simulink model "test_mashinka_mapp_4"  (R2020b)
settings: Solver=ode45  StartTime=0.0  StopTime=20000  RelTol=1e-3  EnableMultiTasking=on
undefined symbols (not defined in the file): CMD_ci_Re_9, CMD_fb, CMD_Firprg_0, CMD_Firprg_1, CMD_gain, CMD_ind_mult, CMD_ind_mult_1, CMD_ind_mult_2, CMD_ind_mult_3, CMD_ind_mult_4, CMD_ind_vol, CMD_ind_vol_1, CMD_ind_vol_2, CMD_ind_vol_3, CMD_ind_vol_4, CMD_nl, CMD_param_0, CMD_pedal, CMD_reset, CMD_shape_0, CMD_step_down, CMD_step_up, ind_mult_0, ind_mult_1, ind_mult_2, ind_mult_3, ind_mult_4, ind_mult_multiplier, num_harm_0, num_pts0, num_str0, num_str1, Res, rom_length
libraries: xbsIndex_r4 x2299
(part 6 of 11)

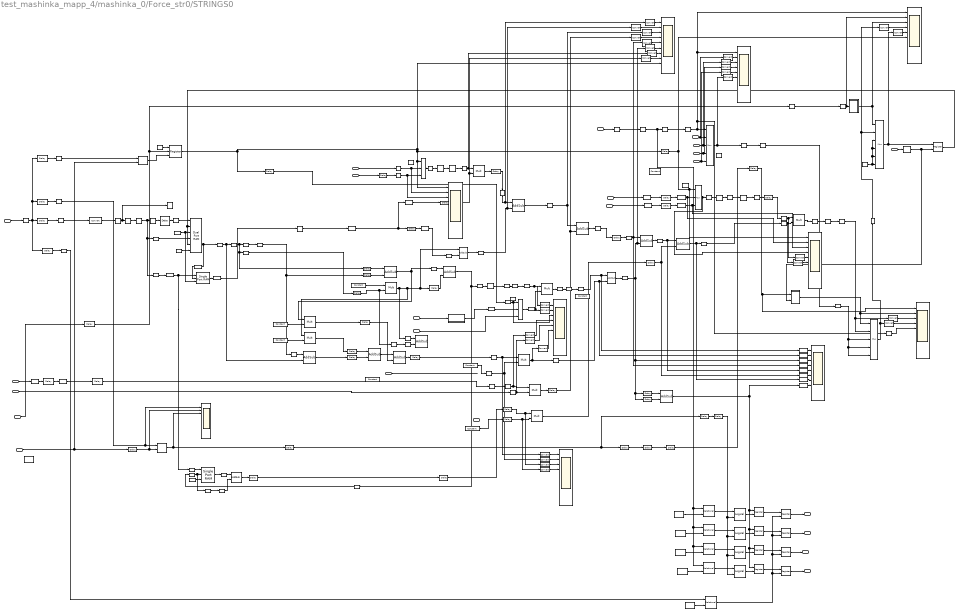
== system test_mashinka_mapp_4/mashinka_0/Force_str0/STRINGS0 ==
  note: Str1[i-2] + Str1[i+2]
  note: 6*Str1[i]
  note: next_plus_last
  note: ff
  note: w20
  note: w41
  note: curr
  note: next
  note: last
  note: prev
  note: decr
  note: e_dt_kvdiv_dx_kv*f_d
  note: e_dt_kvdiv_dx_kv
  note: Str0[i]
  note: 2*Str1[i]
  note: 2*Str1[i] - Str0[i]
  note: Str0[i] *decr_dt
  note: 2*Str1[i] - Str0[i] + Str0[i] *decr_dt
  note: next_plus_last = Str1[i-1] + Str1[i+1];
      |
      | 							str_sd1[i] = next_plus_last - 2*Str1[i];
      |
      | 							str_fd1[i] = Str1[i-2] + Str1[i+2] - 4*(next_plus_last) +6*Str1[i];
  note: 4*next_plus_last
  note: last-last
  note: next-next
  note: 2*curr
  note: str_sd1
  note: str_sd1
  clk : Inport
  rst : Inport  Port=2
  force : Inport  Port=3
  LASTX0 : Inport  Port=4
  Dec : Inport  Port=5
  ddiv : Inport  Port=6
  SHAPE : Inport  Port=7
  Tn : Inport  Port=8
  Disp : Inport  Port=9
  Disp_decr : Inport  Port=10
  sdvig : Inport  Port=11
  damper : Inport  Port=12
  damper_ddiv : Inport  Port=13
  LASTX1 : Inport  Port=14
  ttn_end : Inport  Port=15
  Strob : Inport  Port=16
  Acc : Inport  Port=17
  LASTX2 : Inport  Port=18
  LASTX3 : Inport  Port=19
  A1 : xbsIndex_r4/Dual Port RAM  depth=num_str0*num_point_256 + 130  initVector=zeros  distributed_mem=Block RAM  init_a=0  init_b=0  rst_a=off  rst_b=off  en_a=off  en_b=off  latency=1  write_mode_A=Read Before Write  write_mode_B=Read Before Write  optimize=Speed  dbl_ovrd=off  simulation_type=fast_sim  block_type=dpram
      settings: xl_area=[96 48 48 144 0 0 0]  block_version=VER_STRING_GOES_HERE
  AddSub{,3,8,13..15} (6 alike) : xbsIndex_r4/AddSub  mode=Addition  use_carryin=off  use_carryout=off  en=off  latency=11  precision=Full  arith_type=Unsigned  n_bits=16  bin_pt=14  quantization=Truncate  overflow=Wrap  use_behavioral_HDL=off  hw_selection=DSP48  pipelined=on  dbl_ovrd=off  block_type=addsub
  AddSub{1..2,12,16} (4 alike) : xbsIndex_r4/AddSub  mode=Subtraction  use_carryin=off  use_carryout=off  en=off  latency=11  precision=Full  arith_type=Unsigned  n_bits=16  bin_pt=14  quantization=Truncate  overflow=Wrap  use_behavioral_HDL=off  hw_selection=DSP48  pipelined=on  dbl_ovrd=off  block_type=addsub
  AddSub10 : xbsIndex_r4/AddSub  mode=Addition  use_carryin=off  use_carryout=off  en=off  latency=10  precision=Full  arith_type=Unsigned  n_bits=16  bin_pt=14  quantization=Truncate  overflow=Wrap  use_behavioral_HDL=off  hw_selection=DSP48  pipelined=on  dbl_ovrd=off  block_type=addsub
  AddSub11 : xbsIndex_r4/AddSub  mode=Subtraction  use_carryin=off  use_carryout=off  en=off  latency=9  precision=Full  arith_type=Unsigned  n_bits=16  bin_pt=14  quantization=Truncate  overflow=Wrap  use_behavioral_HDL=off  hw_selection=Fabric  pipelined=off  dbl_ovrd=off  block_type=addsub
  AddSub17 : xbsIndex_r4/AddSub  mode=Subtraction  use_carryin=off  use_carryout=off  en=off  latency=9  precision=Full  arith_type=Unsigned  n_bits=16  bin_pt=14  quantization=Truncate  overflow=Wrap  use_behavioral_HDL=off  hw_selection=Fabric  pipelined=off  dbl_ovrd=off  block_type=addsub
  AddSub9 : xbsIndex_r4/AddSub  mode=Subtraction  use_carryin=off  use_carryout=off  en=off  latency=8  precision=Full  arith_type=Unsigned  n_bits=16  bin_pt=14  quantization=Truncate  overflow=Wrap  use_behavioral_HDL=off  hw_selection=DSP48  pipelined=on  dbl_ovrd=off  block_type=addsub
  B2 : xbsIndex_r4/Single Port RAM  depth=num_str0*num_point_256 + 130  initVector=zeros  distributed_mem=Block RAM  write_mode=Read Before Write  rst=off  init_reg=0  en=off  optimize_latency=off  latency=1  optimize=Speed  dbl_ovrd=off  simulation_type=fast_sim  block_type=spram
      settings: block_version=8.2
  B3 : xbsIndex_r4/Single Port RAM  depth=num_str0*num_point_256 + 130  initVector=zeros  distributed_mem=Block RAM  write_mode=Read Before Write  rst=off  init_reg=0  en=off  optimize_latency=off  latency=1  optimize=Speed  dbl_ovrd=off  simulation_type=fast_sim  block_type=spram
      settings: block_version=8.2
  Constant{1,4,15,17} (4 alike) : xbsIndex_r4/Constant  const=0  gui_display_data_type=Boolean  arith_type=Boolean  n_bits=16  bin_pt=14  preci_type=Single  exp_width=8  frac_width=24  explicit_period=on  period=1  equ=P=C  opselect=C  inp2=PCIN>>17  opr=+  inp1=P  carry=CIN  dbl_ovrd=off  block_type=constant
      settings: block_version=VER_STRING_GOES_HERE
  Constant10 : xbsIndex_r4/Constant  const=2  gui_display_data_type=Fixed-point  arith_type=Unsigned  n_bits=2  bin_pt=0  preci_type=Single  exp_width=8  frac_width=24  explicit_period=on  period=1  equ=P=C  opselect=C  inp2=PCIN>>17  opr=+  inp1=P  carry=CIN  dbl_ovrd=off  block_type=constant
      settings: block_version=VER_STRING_GOES_HERE
  Constant11 : xbsIndex_r4/Constant  const=3  gui_display_data_type=Fixed-point  arith_type=Unsigned  n_bits=2  bin_pt=0  preci_type=Single  exp_width=8  frac_width=24  explicit_period=on  period=1  equ=P=C  opselect=C  inp2=PCIN>>17  opr=+  inp1=P  carry=CIN  dbl_ovrd=off  block_type=constant
      settings: block_version=VER_STRING_GOES_HERE
  Constant12 : xbsIndex_r4/Constant  const=95  gui_display_data_type=Fixed-point  arith_type=Unsigned  n_bits=7  bin_pt=0  preci_type=Single  exp_width=8  frac_width=24  explicit_period=on  period=1  equ=P=C  opselect=C  inp2=PCIN>>17  opr=+  inp1=P  carry=CIN  dbl_ovrd=off  block_type=constant
      settings: block_version=VER_STRING_GOES_HERE
  Constant13 : xbsIndex_r4/Constant  const=201  gui_display_data_type=Fixed-point  arith_type=Unsigned  n_bits=9  bin_pt=0  preci_type=Single  exp_width=8  frac_width=24  explicit_period=on  period=1  equ=P=C  opselect=C  inp2=PCIN>>17  opr=+  inp1=P  carry=CIN  dbl_ovrd=off  block_type=constant
      settings: block_version=VER_STRING_GOES_HERE
  Constant16 : xbsIndex_r4/Constant  const=1  gui_display_data_type=Boolean  arith_type=Boolean  n_bits=16  bin_pt=14  preci_type=Single  exp_width=8  frac_width=24  explicit_period=on  period=1  equ=P=C  opselect=C  inp2=PCIN>>17  opr=+  inp1=P  carry=CIN  dbl_ovrd=off  block_type=constant
      settings: block_version=VER_STRING_GOES_HERE
  Constant18 : xbsIndex_r4/Constant  const=0  gui_display_data_type=Floating-point  arith_type=Floating-point  n_bits=32  bin_pt=0  preci_type=Single  exp_width=8  frac_width=24  explicit_period=on  period=1  equ=P=C  opselect=C  inp2=PCIN>>17  opr=+  inp1=P  carry=CIN  dbl_ovrd=off  block_type=constant
      settings: block_version=VER_STRING_GOES_HERE
  Constant2 : xbsIndex_r4/Constant  const=1  gui_display_data_type=Boolean  arith_type=Boolean  n_bits=16  bin_pt=14  preci_type=Single  exp_width=8  frac_width=24  explicit_period=on  period=1  equ=P=C  opselect=C  inp2=PCIN>>17  opr=+  inp1=P  carry=CIN  dbl_ovrd=off  block_type=constant
      settings: block_version=VER_STRING_GOES_HERE
  Constant3 : xbsIndex_r4/Constant  const=1  gui_display_data_type=Boolean  arith_type=Boolean  n_bits=16  bin_pt=14  preci_type=Single  exp_width=8  frac_width=24  explicit_period=on  period=1  equ=P=C  opselect=C  inp2=PCIN>>17  opr=+  inp1=P  carry=CIN  dbl_ovrd=off  block_type=constant
      settings: block_version=VER_STRING_GOES_HERE
  Constant5 : xbsIndex_r4/Constant  const=0  gui_display_data_type=Floating-point  arith_type=Floating-point  n_bits=16  bin_pt=14  preci_type=Single  exp_width=8  frac_width=24  explicit_period=on  period=1  equ=P=C  opselect=C  inp2=PCIN>>17  opr=+  inp1=P  carry=CIN  dbl_ovrd=off  block_type=constant
      settings: block_version=VER_STRING_GOES_HERE
  Constant6 : xbsIndex_r4/Constant  const=0  gui_display_data_type=Fixed-point  arith_type=Unsigned  n_bits=2  bin_pt=0  preci_type=Single  exp_width=8  frac_width=24  explicit_period=on  period=1  equ=P=C  opselect=C  inp2=PCIN>>17  opr=+  inp1=P  carry=CIN  dbl_ovrd=off  block_type=constant
      settings: block_version=VER_STRING_GOES_HERE
  Constant8 : xbsIndex_r4/Constant  const=1  gui_display_data_type=Fixed-point  arith_type=Unsigned  n_bits=2  bin_pt=0  preci_type=Single  exp_width=8  frac_width=24  explicit_period=on  period=1  equ=P=C  opselect=C  inp2=PCIN>>17  opr=+  inp1=P  carry=CIN  dbl_ovrd=off  block_type=constant
      settings: block_version=VER_STRING_GOES_HERE
  Constant9 : xbsIndex_r4/Constant  const=0  gui_display_data_type=Floating-point  arith_type=Floating-point  n_bits=16  bin_pt=14  preci_type=Single  exp_width=8  frac_width=24  explicit_period=on  period=1  equ=P=C  opselect=C  inp2=PCIN>>17  opr=+  inp1=P  carry=CIN  dbl_ovrd=off  block_type=constant
  Convert{1..4,7,10..28,30..35,37..42} (36 alike) : xbsIndex_r4/Convert  gui_display_data_type=Floating-point  arith_type=Floating-point  n_bits=16  bin_pt=14  float_type=Single  exp_bits=8  fraction_bits=24  quantization=Truncate  overflow=Wrap  en=off  latency=0  pipeline=off  dbl_ovrd=off  block_type=convert
  Convert29 : xbsIndex_r4/Convert  gui_display_data_type=Fixed-point  arith_type="Signed  (2's comp)"  n_bits=25  bin_pt=24  float_type=Single  exp_bits=8  fraction_bits=24  quantization=Truncate  overflow=Wrap  en=off  latency=0  pipeline=off  dbl_ovrd=off  block_type=convert
  Convert36 : xbsIndex_r4/Convert  gui_display_data_type=Fixed-point  arith_type="Signed  (2's comp)"  n_bits=25  bin_pt=24  float_type=Single  exp_bits=8  fraction_bits=24  quantization=Truncate  overflow=Wrap  en=off  latency=0  pipeline=off  dbl_ovrd=off  block_type=convert
  Convert5 : xbsIndex_r4/Convert  gui_display_data_type=Floating-point  arith_type=Floating-point  n_bits=16  bin_pt=14  float_type=Single  exp_bits=8  fraction_bits=24  quantization=Truncate  overflow=Wrap  en=off  latency=6  pipeline=off  dbl_ovrd=off  block_type=convert
  Convert57 : xbsIndex_r4/Convert  gui_display_data_type=Floating-point  arith_type=Floating-point  n_bits=16  bin_pt=14  float_type=Single  exp_bits=8  fraction_bits=24  quantization=Truncate  overflow=Wrap  en=off  latency=8  pipeline=off  dbl_ovrd=off  block_type=convert
  Convert6 : xbsIndex_r4/Convert  gui_display_data_type=Fixed-point  arith_type=Boolean  n_bits=48  bin_pt=48  float_type=Single  exp_bits=8  fraction_bits=24  quantization=Truncate  overflow=Saturate  en=off  latency=0  pipeline=off  dbl_ovrd=off  block_type=convert
      settings: xl_area=[0 0 0 0 0 0 0]  block_version=8.2-EVAL
  Convert8 : xbsIndex_r4/Convert  gui_display_data_type=Floating-point  arith_type=Floating-point  n_bits=16  bin_pt=14  float_type=Single  exp_bits=8  fraction_bits=24  quantization=Truncate  overflow=Wrap  en=off  latency=6  pipeline=off  dbl_ovrd=off  block_type=convert
  Convert9 : xbsIndex_r4/Convert  gui_display_data_type=Fixed-point  arith_type=Unsigned  n_bits=ceil(log2(num_str_12*num_point_256 + 70))  bin_pt=0  float_type=Single  exp_bits=8  fraction_bits=24  quantization=Truncate  overflow=Saturate  en=off  latency=0  pipeline=off  dbl_ovrd=off  block_type=convert
      settings: xl_area=[0 0 0 0 0 0 0]  block_version=8.2-EVAL
  Delay1 : xbsIndex_r4/Delay  rst=off  infoeditControl=Selection of Reset will increase slice count due to use of real FFs and instead of SRLs  en=off  latency=3  reg_retiming=on  dbl_ovrd=off  block_type=delay
      settings: xl_area=[16 32 0 0 0 0 0]  block_version=VER_STRING_GOES_HERE
  Delay10 : xbsIndex_r4/Delay  rst=off  infoeditControl=Selection of Reset will increase slice count due to use of real FFs and instead of SRLs  en=off  latency=17  reg_retiming=on  dbl_ovrd=off  block_type=delay
      settings: xl_area=[2 4 0 4 0 0 0]  block_version=8.2-EVAL
  Delay11 : xbsIndex_r4/Delay  rst=off  infoeditControl=Selection of Reset will increase slice count due to use of real FFs and instead of SRLs  en=off  latency=17  reg_retiming=on  dbl_ovrd=off  block_type=delay
      settings: xl_area=[2 4 0 4 0 0 0]  block_version=8.2-EVAL
  Delay15 : xbsIndex_r4/Delay  rst=off  infoeditControl=Selection of Reset will increase slice count due to use of real FFs and instead of SRLs  en=off  latency=101 + 56  reg_retiming=on  dbl_ovrd=off  block_type=delay
      settings: block_version=VER_STRING_GOES_HERE
  Delay2 : xbsIndex_r4/Delay  rst=off  infoeditControl=Selection of Reset will increase slice count due to use of real FFs and instead of SRLs  en=off  latency=19  reg_retiming=on  dbl_ovrd=off  block_type=delay
      settings: xl_area=[2 4 0 4 0 0 0]  block_version=8.2-EVAL
  Delay{3,5..6,9} (4 alike) : xbsIndex_r4/Delay  rst=off  infoeditControl=Selection of Reset will increase slice count due to use of real FFs and instead of SRLs  en=off  latency=1  reg_retiming=on  dbl_ovrd=off  block_type=delay
      Delay3 settings: xl_area=[16 32 0 0 0 0 0]  block_version=VER_STRING_GOES_HERE
      Delay5 settings: xl_area=[16 32 0 0 0 0 0]  block_version=VER_STRING_GOES_HERE
      Delay6 settings: xl_area=[16 32 0 0 0 0 0]  block_version=VER_STRING_GOES_HERE
      Delay9 settings: infoedit=Hardware notes: A delay line is a chain, each link of which is an SRL16 followed by a flip-flop. If register retiming is enabled, the delay line is a chain of flip-flops.  xl_area=[16 32 0 0 0 0 0]  block_version=VER_STRING_GOES_HERE
  Delay_tn1 : Subsystem
  Logical{,1..3} (4 alike) : xbsIndex_r4/Logical  logical_function=AND  inputs=2  en=off  latency=0  precision=Full  arith_type=Unsigned  n_bits=16  bin_pt=0  align_bp=on  dbl_ovrd=off  block_type=logical
  Mult{,1..2,4..6,10..12} (9 alike) : xbsIndex_r4/Mult  precision=Full  arith_type="Signed  (2's comp)"  n_bits=16  bin_pt=14  quantization=Truncate  overflow=Wrap  en=off  latency=6  use_behavioral_HDL=off  opt=Speed  use_embedded=on  optimum_pipeline=on  pipeline=on  dbl_ovrd=off  use_rpm=on  placement_style=Triangular  block_type=mult
  Mux1 : xbsIndex_r4/Mux  inputs=4  en=off  latency=0  precision=Full  arith_type="Signed  (2's comp)"  n_bits=24  bin_pt=23  quantization=Truncate  overflow=Wrap  dbl_ovrd=off  block_type=mux
      settings: xl_area=[16 0 0 32 0 0 0]  block_version=VER_STRING_GOES_HERE
  Mux2 : xbsIndex_r4/Mux  inputs=2  en=off  latency=0  precision=Full  arith_type="Signed  (2's comp)"  n_bits=24  bin_pt=23  quantization=Truncate  overflow=Wrap  dbl_ovrd=off  block_type=mux
      settings: xl_area=[16 0 0 32 0 0 0]  block_version=VER_STRING_GOES_HERE
  Mux3 : xbsIndex_r4/Mux  inputs=4  en=off  latency=0  precision=Full  arith_type="Signed  (2's comp)"  n_bits=24  bin_pt=23  quantization=Truncate  overflow=Wrap  dbl_ovrd=off  block_type=mux
      settings: xl_area=[16 0 0 32 0 0 0]  block_version=VER_STRING_GOES_HERE
  Mux4 : xbsIndex_r4/Mux  inputs=2  en=off  latency=0  precision=Full  arith_type="Signed  (2's comp)"  n_bits=24  bin_pt=23  quantization=Truncate  overflow=Wrap  dbl_ovrd=off  block_type=mux
      settings: xl_area=[16 0 0 32 0 0 0]  block_version=VER_STRING_GOES_HERE
  Mux5 : xbsIndex_r4/Mux  inputs=2  en=off  latency=0  precision=Full  arith_type="Signed  (2's comp)"  n_bits=24  bin_pt=23  quantization=Truncate  overflow=Wrap  dbl_ovrd=off  block_type=mux
      settings: xl_area=[16 0 0 32 0 0 0]  block_version=VER_STRING_GOES_HERE
  Mux7 : xbsIndex_r4/Mux  inputs=5  en=off  latency=0  precision=Full  arith_type="Signed  (2's comp)"  n_bits=24  bin_pt=23  quantization=Truncate  overflow=Wrap  dbl_ovrd=off  block_type=mux
      settings: xl_area=[16 0 0 32 0 0 0]  block_version=VER_STRING_GOES_HERE
  RSlice6 : xbsIndex_r4/Slice  nbits=1  boolean_output=off  mode=Upper Bit Location + Width  bit1=-1  base1=MSB of Input  bit0=0  base0=LSB of Input  dbl_ovrd=off  block_type=slice
      settings: block_version=VER_STRING_GOES_HERE
  Register : xbsIndex_r4/Register  init=0  rst=on  en=on  dbl_ovrd=off  block_type=register
  Register{2..3,5..6,8..12,16,18,20..24,27..28,30..31,37,42..43,47,61..62,77..81} (31 alike) : xbsIndex_r4/Register  init=0  rst=off  en=off  dbl_ovrd=off  block_type=register
  Register{13..15,17,19,29,32..33} (8 alike) : xbsIndex_r4/Register  init=0  rst=off  en=on  dbl_ovrd=off  block_type=register
  Register4 : xbsIndex_r4/Register  init=0  rst=on  en=off  dbl_ovrd=off  block_type=register
      settings: xl_area=[18 36 0 0 0 0 0]  block_version=VER_STRING_GOES_HERE
  Relational{,2,4,7..8} (5 alike) : xbsIndex_r4/Relational  mode=a=b  op_type=Bool  en=off  latency=1  dbl_ovrd=off  block_type=relational
  Relational1 : xbsIndex_r4/Relational  mode=a=b  op_type=Bool  en=off  latency=0  dbl_ovrd=off  block_type=relational
      settings: xl_area=[3 1 0 6 0 0 0]  block_version=VER_STRING_GOES_HERE
  Relational5 : xbsIndex_r4/Relational  mode=a=b  op_type=Bool  en=off  latency=2  dbl_ovrd=off  block_type=relational
      settings: xl_area=[3 1 0 6 0 0 0]  block_version=VER_STRING_GOES_HERE
  Scope{1..10} (10 alike) : Scope  NumInputPorts=10
  Subsystem1 : Subsystem
  Subsystem2 : Subsystem
  curr1 : xbsIndex_r4/Delay  rst=off  infoeditControl=Selection of Reset will increase slice count due to use of real FFs and instead of SRLs  en=off  latency=16  reg_retiming=on  dbl_ovrd=off  block_type=delay
      settings: xl_area=[17 33 0 33 0 0 0]  block_version=VER_STRING_GOES_HERE
  curr{2..3,5,7,11,13,15..20,23,26,31..34,36..38,40..42,45,48,50,56..57,59..62,67..69,73,77,83,85..88,127,129..130} (46 alike) : xbsIndex_r4/Delay  rst=off  infoeditControl=Selection of Reset will increase slice count due to use of real FFs and instead of SRLs  en=off  latency=1  reg_retiming=on  dbl_ovrd=off  block_type=delay
      curr11 settings: xl_area=[17 33 0 33 0 0 0]  block_version=VER_STRING_GOES_HERE
      curr127 settings: xl_area=[16 32 0 0 0 0 0]  block_version=VER_STRING_GOES_HERE
      curr129 settings: xl_area=[16 32 0 0 0 0 0]  block_version=VER_STRING_GOES_HERE
      curr13 settings: xl_area=[17 33 0 33 0 0 0]  block_version=VER_STRING_GOES_HERE
      curr130 settings: xl_area=[16 32 0 0 0 0 0]  block_version=VER_STRING_GOES_HERE
      curr15 settings: xl_area=[16 32 0 0 0 0 0]  block_version=VER_STRING_GOES_HERE
      curr16 settings: xl_area=[16 32 0 0 0 0 0]  block_version=VER_STRING_GOES_HERE
      curr17 settings: xl_area=[17 33 0 33 0 0 0]  block_version=VER_STRING_GOES_HERE
      curr18 settings: xl_area=[16 32 0 0 0 0 0]  block_version=VER_STRING_GOES_HERE
      curr19 settings: xl_area=[17 33 0 33 0 0 0]  block_version=VER_STRING_GOES_HERE
      curr2 settings: xl_area=[16 32 0 0 0 0 0]  block_version=VER_STRING_GOES_HERE
      curr20 settings: xl_area=[17 33 0 33 0 0 0]  block_version=VER_STRING_GOES_HERE
      curr23 settings: xl_area=[17 33 0 33 0 0 0]  block_version=VER_STRING_GOES_HERE
      curr26 settings: xl_area=[16 32 0 0 0 0 0]  block_version=VER_STRING_GOES_HERE
      curr3 settings: xl_area=[16 32 0 0 0 0 0]  block_version=VER_STRING_GOES_HERE
      curr31 settings: xl_area=[16 32 0 0 0 0 0]  block_version=VER_STRING_GOES_HERE
      curr32 settings: xl_area=[16 32 0 0 0 0 0]  block_version=VER_STRING_GOES_HERE
      curr33 settings: xl_area=[16 32 0 0 0 0 0]  block_version=VER_STRING_GOES_HERE
      curr34 settings: xl_area=[16 32 0 0 0 0 0]  block_version=VER_STRING_GOES_HERE
      curr36 settings: xl_area=[16 32 0 0 0 0 0]  block_version=VER_STRING_GOES_HERE
      curr37 settings: xl_area=[16 32 0 0 0 0 0]  block_version=VER_STRING_GOES_HERE
      curr38 settings: xl_area=[16 32 0 0 0 0 0]  block_version=VER_STRING_GOES_HERE
      curr40 settings: xl_area=[16 32 0 0 0 0 0]  block_version=VER_STRING_GOES_HERE
      curr41 settings: xl_area=[17 33 0 33 0 0 0]  block_version=VER_STRING_GOES_HERE
      curr42 settings: xl_area=[16 32 0 0 0 0 0]  block_version=VER_STRING_GOES_HERE
      curr45 settings: xl_area=[17 33 0 33 0 0 0]  block_version=VER_STRING_GOES_HERE
      curr48 settings: xl_area=[17 33 0 33 0 0 0]  block_version=VER_STRING_GOES_HERE
      curr5 settings: xl_area=[16 32 0 0 0 0 0]  block_version=VER_STRING_GOES_HERE
      curr50 settings: xl_area=[16 32 0 0 0 0 0]  block_version=VER_STRING_GOES_HERE
      curr56 settings: xl_area=[16 32 0 0 0 0 0]  block_version=VER_STRING_GOES_HERE
      curr57 settings: xl_area=[16 32 0 0 0 0 0]  block_version=VER_STRING_GOES_HERE
      curr59 settings: xl_area=[16 32 0 0 0 0 0]  block_version=VER_STRING_GOES_HERE
      curr60 settings: xl_area=[16 32 0 0 0 0 0]  block_version=VER_STRING_GOES_HERE
      curr61 settings: xl_area=[16 32 0 0 0 0 0]  block_version=VER_STRING_GOES_HERE
      curr62 settings: xl_area=[16 32 0 0 0 0 0]  block_version=VER_STRING_GOES_HERE
      curr67 settings: xl_area=[16 32 0 0 0 0 0]  block_version=VER_STRING_GOES_HERE
      curr68 settings: xl_area=[16 32 0 0 0 0 0]  block_version=VER_STRING_GOES_HERE
      curr69 settings: xl_area=[16 32 0 0 0 0 0]  block_version=VER_STRING_GOES_HERE
      curr7 settings: xl_area=[16 32 0 0 0 0 0]  block_version=VER_STRING_GOES_HERE
      curr73 settings: xl_area=[16 32 0 0 0 0 0]  block_version=VER_STRING_GOES_HERE
      curr77 settings: xl_area=[17 33 0 33 0 0 0]  block_version=VER_STRING_GOES_HERE
      curr83 settings: xl_area=[16 32 0 0 0 0 0]  block_version=VER_STRING_GOES_HERE
      curr85 settings: xl_area=[16 32 0 0 0 0 0]  block_version=VER_STRING_GOES_HERE
      curr86 settings: xl_area=[16 32 0 0 0 0 0]  block_version=VER_STRING_GOES_HERE
      curr87 settings: xl_area=[16 32 0 0 0 0 0]  block_version=VER_STRING_GOES_HERE
      curr88 settings: xl_area=[16 32 0 0 0 0 0]  block_version=VER_STRING_GOES_HERE
  curr12 : xbsIndex_r4/Delay  rst=off  infoeditControl=Selection of Reset will increase slice count due to use of real FFs and instead of SRLs  en=off  latency=46  reg_retiming=on  dbl_ovrd=off  block_type=delay
      settings: xl_area=[17 33 0 33 0 0 0]  block_version=VER_STRING_GOES_HERE
  curr{14,27,53..54,76} (5 alike) : xbsIndex_r4/Delay  rst=off  infoeditControl=Selection of Reset will increase slice count due to use of real FFs and instead of SRLs  en=off  latency=5  reg_retiming=on  dbl_ovrd=off  block_type=delay
      curr14 settings: xl_area=[17 33 0 33 0 0 0]  block_version=VER_STRING_GOES_HERE
      curr27 settings: xl_area=[16 32 0 0 0 0 0]  block_version=VER_STRING_GOES_HERE
      curr53 settings: xl_area=[16 32 0 0 0 0 0]  block_version=VER_STRING_GOES_HERE
      curr54 settings: xl_area=[16 32 0 0 0 0 0]  block_version=VER_STRING_GOES_HERE
      curr76 settings: xl_area=[16 32 0 0 0 0 0]  block_version=VER_STRING_GOES_HERE
  curr21 : xbsIndex_r4/Delay  rst=off  infoeditControl=Selection of Reset will increase slice count due to use of real FFs and instead of SRLs  en=off  latency=49 - 7  reg_retiming=on  dbl_ovrd=off  block_type=delay
      settings: xl_area=[17 33 0 33 0 0 0]  block_version=VER_STRING_GOES_HERE
  curr{22,29,43,49} (4 alike) : xbsIndex_r4/Delay  rst=off  infoeditControl=Selection of Reset will increase slice count due to use of real FFs and instead of SRLs  en=off  latency=8  reg_retiming=on  dbl_ovrd=off  block_type=delay
      curr22 settings: xl_area=[17 33 0 33 0 0 0]  block_version=VER_STRING_GOES_HERE
      curr29 settings: xl_area=[16 32 0 0 0 0 0]  block_version=VER_STRING_GOES_HERE
      curr43 settings: xl_area=[16 32 0 0 0 0 0]  block_version=VER_STRING_GOES_HERE
      curr49 settings: xl_area=[16 32 0 0 0 0 0]  block_version=VER_STRING_GOES_HERE
  curr24 : xbsIndex_r4/Delay  rst=off  infoeditControl=Selection of Reset will increase slice count due to use of real FFs and instead of SRLs  en=off  latency=36  reg_retiming=on  dbl_ovrd=off  block_type=delay
      settings: xl_area=[13 26 0 26 0 0 0]  block_version=VER_STRING_GOES_HERE
  curr25 : xbsIndex_r4/Delay  rst=off  infoeditControl=Selection of Reset will increase slice count due to use of real FFs and instead of SRLs  en=off  latency=40  reg_retiming=on  dbl_ovrd=off  block_type=delay
      settings: xl_area=[17 33 0 33 0 0 0]  block_version=VER_STRING_GOES_HERE
  curr28 : xbsIndex_r4/Delay  rst=off  infoeditControl=Selection of Reset will increase slice count due to use of real FFs and instead of SRLs  en=off  latency=7  reg_retiming=on  dbl_ovrd=off  block_type=delay
      settings: xl_area=[16 32 0 0 0 0 0]  block_version=VER_STRING_GOES_HERE
  curr{8,30,51,64} (4 alike) : xbsIndex_r4/Delay  rst=off  infoeditControl=Selection of Reset will increase slice count due to use of real FFs and instead of SRLs  en=off  latency=10  reg_retiming=on  dbl_ovrd=off  block_type=delay
      curr30 settings: xl_area=[16 32 0 0 0 0 0]  block_version=VER_STRING_GOES_HERE
      curr51 settings: xl_area=[16 32 0 0 0 0 0]  block_version=VER_STRING_GOES_HERE
      curr64 settings: xl_area=[17 33 0 33 0 0 0]  block_version=VER_STRING_GOES_HERE
      curr8 settings: xl_area=[17 33 0 33 0 0 0]  block_version=VER_STRING_GOES_HERE
  curr35 : xbsIndex_r4/Delay  rst=off  infoeditControl=Selection of Reset will increase slice count due to use of real FFs and instead of SRLs  en=off  latency=152  reg_retiming=on  dbl_ovrd=off  block_type=delay
      settings: xl_area=[16 32 0 0 0 0 0]  block_version=VER_STRING_GOES_HERE
  curr39 : xbsIndex_r4/Delay  rst=off  infoeditControl=Selection of Reset will increase slice count due to use of real FFs and instead of SRLs  en=off  latency=7  reg_retiming=on  dbl_ovrd=off  block_type=delay
      settings: xl_area=[17 33 0 33 0 0 0]  block_version=VER_STRING_GOES_HERE
  curr4 : xbsIndex_r4/Delay  rst=off  infoeditControl=Selection of Reset will increase slice count due to use of real FFs and instead of SRLs  en=off  latency=28  reg_retiming=on  dbl_ovrd=off  block_type=delay
      settings: xl_area=[13 26 0 26 0 0 0]  block_version=VER_STRING_GOES_HERE
  curr44 : xbsIndex_r4/Delay  rst=off  infoeditControl=Selection of Reset will increase slice count due to use of real FFs and instead of SRLs  en=off  latency=19  reg_retiming=on  dbl_ovrd=off  block_type=delay
      settings: xl_area=[17 33 0 33 0 0 0]  block_version=VER_STRING_GOES_HERE
  curr46 : xbsIndex_r4/Delay  rst=off  infoeditControl=Selection of Reset will increase slice count due to use of real FFs and instead of SRLs  en=off  latency=39  reg_retiming=on  dbl_ovrd=off  block_type=delay
      settings: xl_area=[17 33 0 33 0 0 0]  block_version=VER_STRING_GOES_HERE
  curr47 : xbsIndex_r4/Delay  rst=off  infoeditControl=Selection of Reset will increase slice count due to use of real FFs and instead of SRLs  en=off  latency=102  reg_retiming=on  dbl_ovrd=off  block_type=delay
      settings: xl_area=[17 33 0 33 0 0 0]  block_version=VER_STRING_GOES_HERE
  curr{52,55,63,78} (4 alike) : xbsIndex_r4/Delay  rst=off  infoeditControl=Selection of Reset will increase slice count due to use of real FFs and instead of SRLs  en=off  latency=6  reg_retiming=on  dbl_ovrd=off  block_type=delay
      curr52 settings: xl_area=[16 32 0 0 0 0 0]  block_version=VER_STRING_GOES_HERE
      curr55 settings: xl_area=[16 32 0 0 0 0 0]  block_version=VER_STRING_GOES_HERE
      curr63 settings: xl_area=[16 32 0 0 0 0 0]  block_version=VER_STRING_GOES_HERE
      curr78 settings: xl_area=[17 33 0 33 0 0 0]  block_version=VER_STRING_GOES_HERE
  curr58 : xbsIndex_r4/Delay  rst=off  infoeditControl=Selection of Reset will increase slice count due to use of real FFs and instead of SRLs  en=off  latency=4  reg_retiming=on  dbl_ovrd=off  block_type=delay
      settings: xl_area=[17 33 0 33 0 0 0]  block_version=VER_STRING_GOES_HERE
  curr6 : xbsIndex_r4/Delay  rst=off  infoeditControl=Selection of Reset will increase slice count due to use of real FFs and instead of SRLs  en=off  latency=2  reg_retiming=on  dbl_ovrd=off  block_type=delay
      settings: xl_area=[16 32 0 0 0 0 0]  block_version=VER_STRING_GOES_HERE
  curr65 : xbsIndex_r4/Delay  rst=off  infoeditControl=Selection of Reset will increase slice count due to use of real FFs and instead of SRLs  en=off  latency=39  reg_retiming=on  dbl_ovrd=off  block_type=delay
      settings: xl_area=[17 33 0 33 0 0 0]  block_version=VER_STRING_GOES_HERE
  curr70 : xbsIndex_r4/Delay  rst=off  infoeditControl=Selection of Reset will increase slice count due to use of real FFs and instead of SRLs  en=off  latency=23  reg_retiming=on  dbl_ovrd=off  block_type=delay
      settings: xl_area=[16 32 0 0 0 0 0]  block_version=VER_STRING_GOES_HERE
  curr72 : xbsIndex_r4/Delay  rst=off  infoeditControl=Selection of Reset will increase slice count due to use of real FFs and instead of SRLs  en=off  latency=3  reg_retiming=on  dbl_ovrd=off  block_type=delay
      settings: xl_area=[16 32 0 0 0 0 0]  block_version=VER_STRING_GOES_HERE
  curr74 : xbsIndex_r4/Delay  rst=off  infoeditControl=Selection of Reset will increase slice count due to use of real FFs and instead of SRLs  en=off  latency=2  reg_retiming=on  dbl_ovrd=off  block_type=delay
      settings: xl_area=[16 32 0 0 0 0 0]  block_version=VER_STRING_GOES_HERE
  curr75 : xbsIndex_r4/Delay  rst=off  infoeditControl=Selection of Reset will increase slice count due to use of real FFs and instead of SRLs  en=off  latency=25  reg_retiming=on  dbl_ovrd=off  block_type=delay
      settings: xl_area=[16 32 0 0 0 0 0]  block_version=VER_STRING_GOES_HERE
  curr79 : xbsIndex_r4/Delay  rst=off  infoeditControl=Selection of Reset will increase slice count due to use of real FFs and instead of SRLs  en=off  latency=50  reg_retiming=on  dbl_ovrd=off  block_type=delay
      settings: xl_area=[16 32 0 0 0 0 0]  block_version=VER_STRING_GOES_HERE
  curr80 : xbsIndex_r4/Delay  rst=off  infoeditControl=Selection of Reset will increase slice count due to use of real FFs and instead of SRLs  en=off  latency=3  reg_retiming=on  dbl_ovrd=off  block_type=delay
      settings: xl_area=[16 32 0 0 0 0 0]  block_version=VER_STRING_GOES_HERE
  curr82 : xbsIndex_r4/Delay  rst=off  infoeditControl=Selection of Reset will increase slice count due to use of real FFs and instead of SRLs  en=off  latency=100  reg_retiming=on  dbl_ovrd=off  block_type=delay
      settings: xl_area=[16 32 0 0 0 0 0]  block_version=VER_STRING_GOES_HERE
  curr84 : xbsIndex_r4/Delay  rst=off  infoeditControl=Selection of Reset will increase slice count due to use of real FFs and instead of SRLs  en=off  latency=7  reg_retiming=on  dbl_ovrd=off  block_type=delay
      settings: xl_area=[16 32 0 0 0 0 0]  block_version=VER_STRING_GOES_HERE
  curr9 : xbsIndex_r4/Delay  rst=off  infoeditControl=Selection of Reset will increase slice count due to use of real FFs and instead of SRLs  en=off  latency=54  reg_retiming=on  dbl_ovrd=off  block_type=delay
      settings: xl_area=[16 32 0 0 0 0 0]  block_version=VER_STRING_GOES_HERE
  float {1,3,5,11} (4 alike) : xbsIndex_r4/Constant  const=0  gui_display_data_type=Floating-point  arith_type=Floating-point  n_bits=32  bin_pt=0  preci_type=Single  exp_width=8  frac_width=24  explicit_period=on  period=1  equ=P=C  opselect=C  inp2=PCIN>>17  opr=+  inp1=P  carry=CIN  dbl_ovrd=off  block_type=constant
      settings: block_version=VER_STRING_GOES_HERE
  float 2 : xbsIndex_r4/Constant  const=2  gui_display_data_type=Floating-point  arith_type=Floating-point  n_bits=32  bin_pt=0  preci_type=Single  exp_width=8  frac_width=24  explicit_period=on  period=1  equ=P=C  opselect=C  inp2=PCIN>>17  opr=+  inp1=P  carry=CIN  dbl_ovrd=off  block_type=constant
      settings: block_version=VER_STRING_GOES_HERE
  float 8 : xbsIndex_r4/Constant  const=4  gui_display_data_type=Floating-point  arith_type=Floating-point  n_bits=32  bin_pt=0  preci_type=Single  exp_width=8  frac_width=24  explicit_period=on  period=1  equ=P=C  opselect=C  inp2=PCIN>>17  opr=+  inp1=P  carry=CIN  dbl_ovrd=off  block_type=constant
      settings: block_version=VER_STRING_GOES_HERE
  float 9 : xbsIndex_r4/Constant  const=3  gui_display_data_type=Floating-point  arith_type=Floating-point  n_bits=32  bin_pt=0  preci_type=Single  exp_width=8  frac_width=24  explicit_period=on  period=1  equ=P=C  opselect=C  inp2=PCIN>>17  opr=+  inp1=P  carry=CIN  dbl_ovrd=off  block_type=constant
      settings: block_version=VER_STRING_GOES_HERE
  prg1 : xbsIndex_r4/Delay  rst=off  infoeditControl=Selection of Reset will increase slice count due to use of real FFs and instead of SRLs  en=off  latency=31  reg_retiming=on  dbl_ovrd=off  block_type=delay
      settings: block_version=8.2-EVAL
  prg2 : xbsIndex_r4/Delay  rst=off  infoeditControl=Selection of Reset will increase slice count due to use of real FFs and instead of SRLs  en=off  latency=9  reg_retiming=on  dbl_ovrd=off  block_type=delay
      settings: block_version=8.2-EVAL
  prg3 : xbsIndex_r4/Delay  rst=off  infoeditControl=Selection of Reset will increase slice count due to use of real FFs and instead of SRLs  en=off  latency=6  reg_retiming=on  dbl_ovrd=off  block_type=delay
      settings: block_version=8.2-EVAL
  prg4 : xbsIndex_r4/Delay  rst=off  infoeditControl=Selection of Reset will increase slice count due to use of real FFs and instead of SRLs  en=off  latency=9  reg_retiming=on  dbl_ovrd=off  block_type=delay
      settings: block_version=8.2-EVAL
  Force_nota0 : Outport  VectorParamsAs1DForOutWhenUnconnected=off
  Force_nota1 : Outport  Port=2  VectorParamsAs1DForOutWhenUnconnected=off
  Force_nota2 : Outport  Port=3  VectorParamsAs1DForOutWhenUnconnected=off
  Force_nota3 : Outport  Port=4  VectorParamsAs1DForOutWhenUnconnected=off
  wires:
  Register19/1 -> Force_nota0/1
  Register13/1 -> Register19/1
  curr72/1 -> Register12/1
  Subsystem2/1(Out1) -> Scope5/2, Mux3/1
  rst/1 -> Convert6/1
  LASTX1/1 -> Convert34/1, Mux1/3
  curr78/1 -> AddSub15/2
  curr77/1 -> AddSub15/1
  curr76/1 -> Mult10/2, Convert4/1
  ttn_end/1 -> Mux5/3
  Mux5/1 -> curr76/1
  Delay_tn1/1(Out1) -> curr67/1
  curr67/1 -> Mux5/2
  curr12/1 -> curr32/1
  Mux3/1 -> Convert17/1, curr16/1
  curr40/1 -> Convert5/1
  SHAPE/1 -> curr62/1
  curr64/1 -> curr1/1
  AddSub1/1 -> curr72/1, curr68/1
  Tn/1 -> Delay_tn1/1(Tn)
  float 11/1 -> curr14/1
  Disp/1 -> ?
  curr7/1 -> curr70/1
  curr80/1 -> Mult4/2, Convert27/1
  curr30/1 -> curr26/1
  curr26/1 -> Mult10/1, Convert3/1
  curr88/1 -> Convert23/1, AddSub10/2, curr77/1, curr78/1, Convert12/1
  curr37/1 -> Convert32/1, AddSub11/1
  curr74/1 -> curr127/1
  curr73/1 -> curr74/1
  Mult10/1 -> curr73/1
  curr69/1 -> curr30/1
  Convert57/1 -> curr69/1
  curr68/1 -> Convert57/1
  curr65/1 -> curr11/1
  Register31/1 -> Relational1/1
  Constant2/1 -> Register/1
  Convert29/1 -> curr40/1
  curr39/1 -> Convert21/1, AddSub8/2
  Convert36/1 -> Convert8/1
  curr59/1 -> Convert29/1
  AddSub8/1 -> curr33/1
  curr14/1 -> Convert30/1, Mult5/2
  curr13/1 -> Convert28/1, Mult5/1
  curr23/1 -> Convert36/1
  Convert5/1 -> curr60/1
  AddSub11/1 -> Convert41/1, curr38/1
  curr45/1 -> AddSub11/2, Convert40/1
  AddSub10/1 -> curr37/1
  curr44/1 -> curr42/1
  Mult6/1 -> curr39/1
  AddSub13/1 -> curr57/1
  curr63/1 -> curr2/1
  curr29/1 -> curr56/1
  Mult1/1 -> curr29/1
  AddSub2/1 -> curr50/1
  curr28/1 -> AddSub2/2
  Register37/1 -> curr28/1
  curr52/1 -> Convert25/1, Mult1/2
  Convert8/1 -> curr58/1
  curr27/1 -> AddSub1/2
  AddSub/1 -> Mult11/1, curr5/1
  Mult/1 -> curr83/1, Mult12/1, curr27/1, AddSub2/1
  curr54/1 -> AddSub/2
  curr53/1 -> AddSub/1
  curr55/1 -> curr84/1, Mult/2
  float 2/1 -> Mult/1
  Delay6/1 -> Delay15/1
  Delay5/1 -> Delay1/1, RSlice6/1
  Delay3/1 -> Delay6/1, Register80/1, Register81/1
  Register3/1 -> Register16/1, curr53/1, Register21/1
  Register16/1 -> curr55/1
  B3/1 -> Register28/1
  ddiv/1 -> Register61/1
  Delay2/1 -> Register47/1
  Register47/1 -> Delay10/1
  prg1/1 -> Register78/1
  clk/1 -> Register77/1
  A1/2 -> Register8/1, Register9/1
  Register21/1 -> Register22/1
  curr6/1 -> Register37/1
  Delay9/1 -> Register23/1
  Register22/1 -> Register2/1, curr54/1
  Constant16/1 -> B3/3, A1/3
  Register8/1 -> B3/2
  Delay1/1 -> Delay3/1
  Delay15/1 -> Register79/1
  Register28/1 -> Delay9/1
  Register5/1 -> Register6/1, B3/1
  Constant17/1 -> A1/6
  Convert9/1 -> Delay5/1
  Convert6/1 -> Register4/2, Subsystem2/2(In2)
  curr4/1 -> Register62/1
  Register10/1 -> Delay2/1
  Register11/1 -> curr52/1
  Register23/1 -> Register11/1, curr6/1
  Register61/1 -> curr4/1
  Register77/1 -> prg4/1, prg3/1, prg2/1, prg1/1
  Register78/1 -> Convert9/1
  Register79/1 -> A1/1
  Register80/1 -> A1/4
  Register81/1 -> Register5/1
  Relational5/1 -> Scope3/3, curr21/1
  curr17/1 -> curr19/1
  curr19/1 -> curr20/1
  prg2/1 -> Register30/1
  damper/1 -> curr22/1
  sdvig/1 -> Relational1/2, curr8/1
  curr20/1 -> curr47/1
  Mux2/1 -> curr23/1
  prg3/1 -> Register31/1
  curr24/1 -> Register43/1
  Register42/1 -> curr24/1
  damper_ddiv/1 -> Register42/1
  curr33/1 -> curr44/1
  curr5/1 -> AddSub1/1
  curr50/1 -> Convert19/1, AddSub13/2
  curr56/1 -> Convert18/1, AddSub13/1
  curr57/1 -> AddSub8/1, Convert20/1
  curr58/1 -> Convert24/1, Mult1/1
  curr60/1 -> curr46/1
  curr62/1 -> Mult6/2, Convert14/1
  prg4/1 -> Register18/1
  AddSub9/1 -> curr88/1
  curr127/1 -> Convert10/1, AddSub9/1
  Mult4/1 -> Convert15/1, curr129/1
  curr129/1 -> Convert11/1, AddSub9/2
  curr130/1 -> Convert26/1, Mult4/1
  float 8/1 -> Mult11/2
  float 9/1 -> Mult12/2
  Register2/1 -> AddSub3/1
  AddSub3/1 -> curr43/1
  Register9/1 -> AddSub3/2, Register3/1
  Mult12/1 -> curr36/1
  curr43/1 -> AddSub14/2
  AddSub14/1 -> AddSub16/1
  Mult11/1 -> curr49/1
  curr36/1 -> AddSub14/1
  curr49/1 -> AddSub16/2
  AddSub16/1 -> curr51/1
  curr51/1 -> curr130/1
  force/1 -> Register10/1
  Register4/1 -> A1/5, A1/2
  Constant18/1 -> Mux7/6, Mux7/4, Mux7/3, Mux7/5
  curr15/1 -> Scope1/2, Subsystem1/1(In1)
  curr35/1 -> curr15/1
  Mux7/1 -> Convert2/1, Register4/1
  curr16/1 -> Convert1/1, Mux7/2
  Constant3/1 -> B2/3
  Register6/1 -> B2/1
  Register12/1 -> Register27/1, B2/2
  Register20/1 -> AddSub12/1
  Register24/1 -> AddSub12/2
  B2/1 -> Register20/1
  Register27/1 -> Register24/1
  AddSub12/1 -> curr64/1
  curr1/1 -> curr13/1
  Mult5/1 -> curr45/1
  curr38/1 -> curr3/1
  Mult2/1 -> curr31/1
  curr18/1 -> Mux3/3, Mux3/5, Mux3/4
  curr31/1 -> curr9/1
  curr61/1 -> Mult2/1, Convert7/1
  Subsystem1/1(Out1) -> Mux7/1, Scope1/3
  AddSub15/1 -> Register13/1, Register14/1, Register15/1, Register17/1, Convert42/1
  curr32/1 -> Scope2/3, Mux5/1
  curr83/1 -> AddSub17/1
  curr84/1 -> curr85/1
  curr85/1 -> AddSub17/2
  curr46/1 -> curr61/1
  curr70/1 -> curr18/1
  curr21/1 -> curr65/1, curr17/1
  curr9/1 -> curr34/1
  Convert1/1 -> Scope1/4
  Convert2/1 -> Scope1/5
  Convert3/1 -> Scope2/1
  Convert4/1 -> Scope2/2
  curr25/1 -> Scope4/1, Mux4/1, Scope1/6
  Register62/1 -> Scope4/2, Mux4/2
  curr2/1 -> Convert13/1, Mult6/1
  Register43/1 -> Scope4/3, Mux4/3
  Mux4/1 -> Scope4/4, curr59/1
  Convert13/1 -> Scope2/4
  Convert14/1 -> Scope2/5
  Convert15/1 -> Scope2/6
  Convert16/1 -> Scope5/3
  curr34/1 -> Convert16/1, Mux3/2
  curr47/1 -> Scope5/1, Subsystem2/1(In1)
  Convert17/1 -> Scope5/4
  Register30/1 -> Scope3/1, Relational5/1
  Relational1/1 -> Register/3
  Convert18/1 -> Scope6/1
  Convert19/1 -> Scope6/2
  Convert20/1 -> Scope6/3
  Convert21/1 -> Scope6/4
  curr42/1 -> Convert31/1, Convert22/1, AddSub10/1
  Convert22/1 -> Scope6/5
  Convert23/1 -> Scope6/6
  Convert24/1 -> Scope6/7
  Convert25/1 -> Scope6/8
  Strob/1 -> Delay11/1
  Delay10/1 -> curr63/1
  Delay11/1 -> Register/2, curr35/1
  Convert26/1 -> Scope7/1
  Convert27/1 -> Scope7/2
  Convert28/1 -> Scope7/3
  Convert30/1 -> Scope7/4
  curr11/1 -> Logical/2, Logical1/2, Logical2/2, Logical3/2
  Dec/1 -> curr41/1
  curr22/1 -> curr48/1
  curr3/1 -> Convert38/1, Mult2/2
  Convert7/1 -> Scope4/5
  Convert38/1 -> Scope4/6
  curr41/1 -> Scope9/2, Mux2/2
  curr48/1 -> Scope9/3, Mux2/3
  Register/1 -> curr25/1, Mux2/1, Scope9/1, Scope6/9, curr12/1
  LASTX2/1 -> Convert35/1, Mux1/4
  curr75/1 -> Scope5/5
  Acc/1 -> curr82/1
  curr79/1 -> curr87/1
  curr82/1 -> curr86/1
  curr86/1 -> Relational/1, Relational2/1, Relational4/1, Relational7/1, curr79/1
  Constant6/1 -> Relational/2
  Constant8/1 -> Relational2/2
  Constant11/1 -> Relational7/2
  Constant10/1 -> Relational4/2
  Relational/1 -> Logical/1
  Relational2/1 -> Logical1/1
  Relational4/1 -> Logical2/1
  Relational7/1 -> Logical3/1
  Logical3/1 -> Register17/2
  Logical2/1 -> Register15/2
  Logical1/1 -> Register14/2
  Logical/1 -> Register13/2
  Register18/1 -> Relational8/1
  Constant12/1 -> Relational8/2
  Relational8/1 -> Register33/2, Register32/2, Register29/2, Register19/2
  Register17/1 -> Register33/1
  Register15/1 -> Register32/1
  Register14/1 -> Register29/1
  Register33/1 -> Force_nota3/1
  Register32/1 -> Force_nota2/1
  Register29/1 -> Force_nota1/1
  curr87/1 -> curr75/1, Scope10/1, Scope1/1, Mux1/1
  Convert33/1 -> Scope10/2
  LASTX0/1 -> Convert33/1, Mux1/2
  LASTX3/1 -> Convert37/1, Mux1/5
  Convert34/1 -> Scope10/3
  Convert35/1 -> Scope10/4
  Convert37/1 -> Scope10/5
  Mux1/1 -> Convert39/1, curr7/1
  Convert39/1 -> Scope10/6
  curr8/1 -> Scope3/2, Relational5/2
  Convert10/1 -> Scope8/1
  Convert11/1 -> Scope8/2
  Convert12/1 -> Scope8/3
  Convert31/1 -> Scope8/4
  Convert32/1 -> Scope8/5
  Convert40/1 -> Scope8/6
  float 3/1 -> curr80/1
  Convert41/1 -> Scope8/7
  Convert42/1 -> Scope8/8

== system test_mashinka_mapp_4/mashinka_0/Force_str0/strob ==
  In1 : Inport
  Convert : xbsIndex_r4/Convert  gui_display_data_type=Boolean  arith_type=Boolean  n_bits=16  bin_pt=14  float_type=Single  exp_bits=8  fraction_bits=24  quantization=Truncate  overflow=Wrap  en=off  latency=0  pipeline=off  dbl_ovrd=off  block_type=convert
      settings: block_version=10.1.1
  Delay9 : xbsIndex_r4/Delay  rst=off  infoeditControl=Selection of Reset will increase slice count due to use of real FFs and instead of SRLs  en=off  latency=1  reg_retiming=on  dbl_ovrd=off  block_type=delay
      settings: infoedit=Hardware notes: A delay line is a chain, each link of which is an SRL16 followed by a flip-flop. If register retiming is enabled, the delay line is a chain of flip-flops.  xl_area=[2 4 0 4 0 0 0]  block_version=8.2-EVAL
  Logical1 : xbsIndex_r4/Logical  logical_function=XOR  inputs=2  en=off  latency=0  precision=User Defined  arith_type=Unsigned  n_bits=1  bin_pt=0  align_bp=on  dbl_ovrd=off  block_type=logical
      settings: block_version=10.1.1
  Out1 : Outport  VectorParamsAs1DForOutWhenUnconnected=off
  wires:
  Convert/1 -> Out1/1
  In1/1 -> Logical1/1, Delay9/1
  Delay9/1 -> Logical1/2
  Logical1/1 -> Convert/1
